simulink model "PID_joint4"  (R2017b)
settings: Solver=VariableStepAuto  StartTime=0.0  StopTime=0.37281  RelTol=1e-3
settings Model: Creator=84935  LastModifiedBy=84935

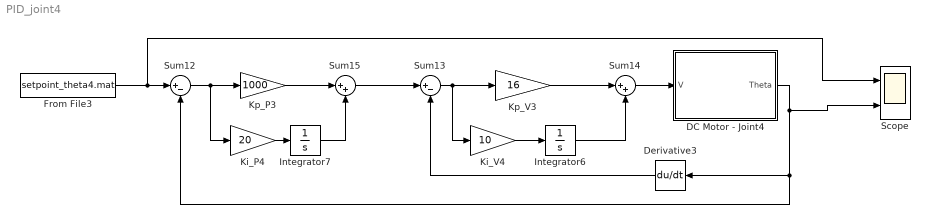
== system PID_joint4 ==
  DC Motor - Joint4 : Subsystem  mask{L=0.012342, R=3.2645, Ki=1.1895, Jeff=0.01829, Beff=0.019, Kb=1.1895, N=50}
  Derivative3 : Derivative
  From File3 : FromFile  FileName=setpoint_theta4.mat  SampleTime=0
  Integrator6 : Integrator
  Integrator7 : Integrator
  Ki_P4 : Gain  Gain=20
  Ki_V4 : Gain  Gain=10
  Kp_P3 : Gain  Gain=1000
  Kp_V3 : Gain  Gain=16
  Scope : Scope  NumInputPorts=2
  Sum12 : Sum  Inputs=|+-
  Sum13 : Sum  Inputs=|+-
  Sum14 : Sum  Inputs=|++
  Sum15 : Sum  Inputs=|++
  wires:
  Integrator7/1 -> Sum15/2
  Ki_P4/1 -> Integrator7/1
  Kp_V3/1 -> Sum14/1
  From File3/1 -> Scope/1, Sum12/1
  Integrator6/1 -> Sum14/2
  Kp_P3/1 -> Sum15/1
  Sum14/1 -> DC Motor - Joint4/1(V)
  Sum15/1 -> Sum13/1
  Derivative3/1 -> Sum13/2
  Sum12/1 -> Ki_P4/1, Kp_P3/1
  DC Motor - Joint4/1(Theta) -> Scope/2, Sum12/2, Derivative3/1
  Sum13/1 -> Kp_V3/1, Ki_V4/1
  Ki_V4/1 -> Integrator6/1

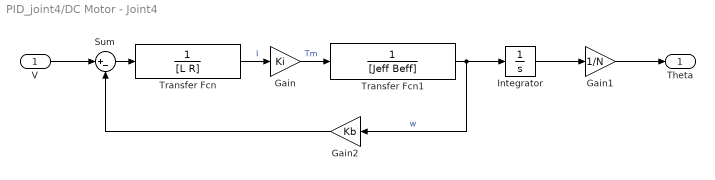
== system PID_joint4/DC Motor - Joint4 ==
  V : Inport
  Gain : Gain  Gain=Ki
  Gain1 : Gain  Gain=1/N
  Gain2 : Gain  Gain=Kb
  Integrator : Integrator
  Sum : Sum  Inputs=|+-
  Transfer Fcn : TransferFcn  Denominator=[L R]
  Transfer Fcn1 : TransferFcn  Denominator=[Jeff Beff]
  Theta : Outport
  wires:
  Integrator/1 -> Gain1/1
  Transfer Fcn1/1 -> Integrator/1, Gain2/1  "w"
  V/1 -> Sum/1
  Gain2/1 -> Sum/2
  Gain/1 -> Transfer Fcn1/1  "Tm"
  Gain1/1 -> Theta/1
  Sum/1 -> Transfer Fcn/1
  Transfer Fcn/1 -> Gain/1  "I"
